simulink model "ex5"  (Simulink 8.5)
settings: Solver=ode3  StartTime=0.0  StopTime=60  FixedStep=0.001  RelTol=1e-3
settings Model: Creator=Dinis  LastModifiedBy=Dinis  CovModelRefEnable=off
settings DataIOCC: LimitDataPoints=off  SaveFormat=Dataset  SignalLoggingSaveFormat=Dataset
settings OptimizationCC: ExpressionDepthLimit=128
settings DebuggingCC: UnderspecifiedInitializationDetection=Simplified  MergeDetectMultiDrivingBlocksExec=error  FcnCallInpInsideContextMsg=EnableAllAsError  StateNameClashWarn=none
settings HardwareCC: ProdBitPerPointer=64  ProdLargestAtomicFloat=Float  ProdIntDivRoundTo=Zero  ProdEndianess=LittleEndian  ProdHWDeviceType=Specified
settings ModelReferenceCC: PropagateSignalLabelsOutOfModel=on
settings GRTTargetCC: CombineOutputUpdateFcns=on  GRTInterface=off

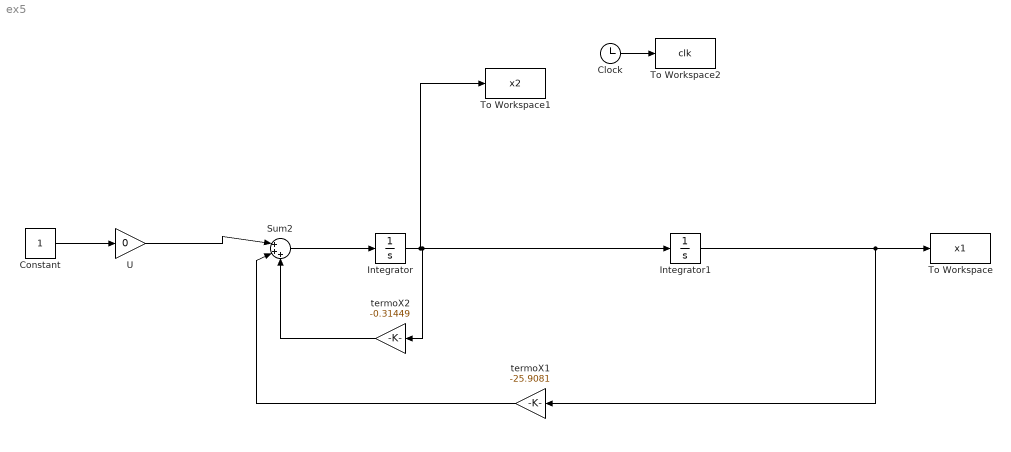
== system ex5 ==
  Clock : Clock
  Constant : Constant
  Integrator : Integrator
  Integrator1 : Integrator  InitialCondition=pi/4
  Sum2 : Sum  Inputs=|+++
  To Workspace : ToWorkspace  VariableName=x1  SampleTime=-1
  To Workspace1 : ToWorkspace  VariableName=x2  SampleTime=-1
  To Workspace2 : ToWorkspace  VariableName=clk  SampleTime=-1
  U : Gain  Gain=0
  termoX1 : Gain  Gain=-25.9081
  termoX2 : Gain  Gain=-0.31449
  wires:
  Integrator1/1 -> To Workspace/1, termoX1/1
  termoX1/1 -> Sum2/2
  Sum2/1 -> Integrator/1
  termoX2/1 -> Sum2/3
  Integrator/1 -> Integrator1/1, termoX2/1, To Workspace1/1
  U/1 -> Sum2/1
  Constant/1 -> U/1
  Clock/1 -> To Workspace2/1
